simulink subsystem "low_level_mapper"  (R2020a)
settings: Solver=VariableStepAuto  StartTime=0.0  StopTime=10.0  RelTol=1e-3
values from neighbouring files (symbols this model uses):
  com_delay = 0.04    [init_conditions.m]
  g = 9.81    [init_conditions.m]
  m = (m_qc+0.006)*4 + m_main    (= 0.156)    [init_conditions.m]
undefined symbols (not defined in the file or in its folder): X, Y, Z
libraries: sm_lib x8, nesl_utility x8, simulink_extras x4
settings Model: Creator=Paul  LastModifiedBy=Paul

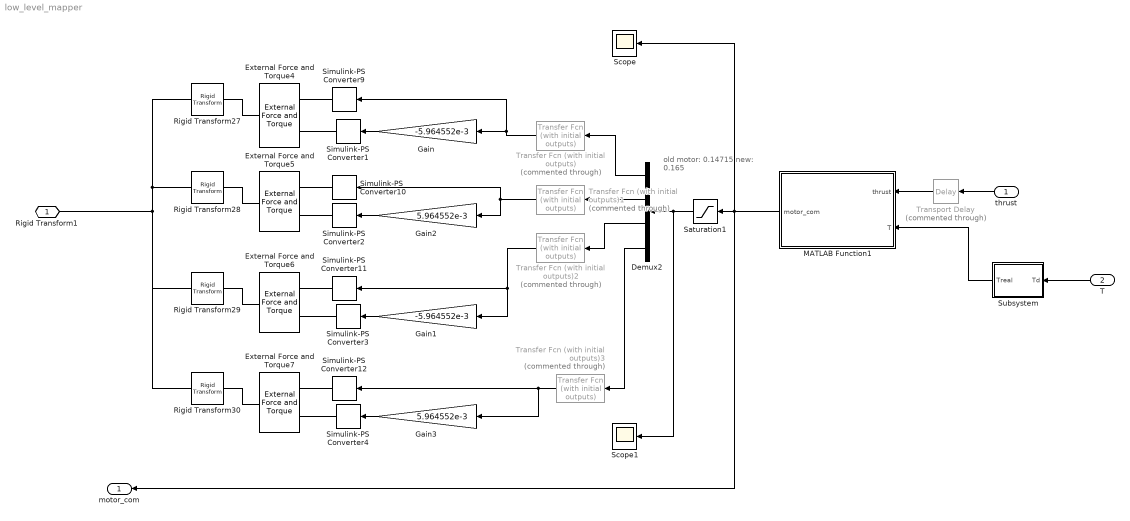
== system low_level_mapper ==
  note: old motor: 0.14715
      | new: 0.165
  thrust : Inport
  T : Inport  Port=2
  Demux2 : Demux
  External Force and Torque{4..7} (4 alike) : sm_lib/Forces and Torques/External Force and Torque  ForceResolutionFrame=AttachedFrame  EnableForceX=off  EnableForceY=off  EnableForceZ=on  EnableForce=off  TorqueResolutionFrame=AttachedFrame  EnableTorqueX=off  EnableTorqueY=off  EnableTorqueZ=on  EnableTorque=off
  Gain : Gain  Gain=-5.964552e-3
  Gain1 : Gain  Gain=-5.964552e-3
  Gain2 : Gain  Gain=5.964552e-3
  Gain3 : Gain  Gain=5.964552e-3
  MATLAB Function1 : MATLAB Function  TreatAsAtomicUnit=on
  Rigid Transform27 : sm_lib/Frames and Transforms/Rigid Transform  TranslationMethod=Cartesian  TranslationStandardOffset=0.4  TranslationLengthUnit=m  TranslationStandardAxis=+X  TranslationCartesianOffset=[0.03165 0.03165 0]  TranslationROffset=0  TranslationROffsetUnits=m  TranslationZOffset=0  TranslationZOffsetUnits=m  TranslationThetaOffset=0  TranslationThetaOffsetUnits=deg  RotationMethod=None  RotationAngleUnits=deg  RotationStandardAxis=+X  RotationAngle=90  RotationArbitraryAxis=[0 0 1]  FollAlignAxisA=+X  BaseAlignAxisA=+Y  FollAlignAxisB=+Y  BaseAlignAxisB=+Z  RotationSequenceAxes=FollowerAxes  RotationSequence=XYX  RotationSequenceAngles=[0 0 0]  RotationSequenceAnglesUnits=deg  RotationMatrix=[1 0 0; 0 1 0; 0 0 1]
  Rigid Transform28 : sm_lib/Frames and Transforms/Rigid Transform  TranslationMethod=Cartesian  TranslationStandardOffset=0.4  TranslationLengthUnit=m  TranslationStandardAxis=+X  TranslationCartesianOffset=[0.03165 -0.03165 0]  TranslationROffset=0  TranslationROffsetUnits=m  TranslationZOffset=0  TranslationZOffsetUnits=m  TranslationThetaOffset=0  TranslationThetaOffsetUnits=deg  RotationMethod=None  RotationAngleUnits=deg  RotationStandardAxis=+X  RotationAngle=90  RotationArbitraryAxis=[0 0 1]  FollAlignAxisA=+X  BaseAlignAxisA=+Y  FollAlignAxisB=+Y  BaseAlignAxisB=+Z  RotationSequenceAxes=FollowerAxes  RotationSequence=XYX  RotationSequenceAngles=[0 0 0]  RotationSequenceAnglesUnits=deg  RotationMatrix=[1 0 0; 0 1 0; 0 0 1]
  Rigid Transform29 : sm_lib/Frames and Transforms/Rigid Transform  TranslationMethod=Cartesian  TranslationStandardOffset=0.4  TranslationLengthUnit=m  TranslationStandardAxis=+X  TranslationCartesianOffset=[-0.03165 -0.03165 0]  TranslationROffset=0  TranslationROffsetUnits=m  TranslationZOffset=0  TranslationZOffsetUnits=m  TranslationThetaOffset=0  TranslationThetaOffsetUnits=deg  RotationMethod=None  RotationAngleUnits=deg  RotationStandardAxis=+X  RotationAngle=90  RotationArbitraryAxis=[0 0 1]  FollAlignAxisA=+X  BaseAlignAxisA=+Y  FollAlignAxisB=+Y  BaseAlignAxisB=+Z  RotationSequenceAxes=FollowerAxes  RotationSequence=XYX  RotationSequenceAngles=[0 0 0]  RotationSequenceAnglesUnits=deg  RotationMatrix=[1 0 0; 0 1 0; 0 0 1]
  Rigid Transform30 : sm_lib/Frames and Transforms/Rigid Transform  TranslationMethod=Cartesian  TranslationStandardOffset=0.4  TranslationLengthUnit=m  TranslationStandardAxis=+X  TranslationCartesianOffset=[-0.03165 0.03165 0]  TranslationROffset=0  TranslationROffsetUnits=m  TranslationZOffset=0  TranslationZOffsetUnits=m  TranslationThetaOffset=0  TranslationThetaOffsetUnits=deg  RotationMethod=None  RotationAngleUnits=deg  RotationStandardAxis=+X  RotationAngle=90  RotationArbitraryAxis=[0 0 1]  FollAlignAxisA=+X  BaseAlignAxisA=+Y  FollAlignAxisB=+Y  BaseAlignAxisB=+Z  RotationSequenceAxes=FollowerAxes  RotationSequence=XYX  RotationSequenceAngles=[0 0 0]  RotationSequenceAnglesUnits=deg  RotationMatrix=[1 0 0; 0 1 0; 0 0 1]
  Saturation1 : Saturate  UpperLimit=0.17  LowerLimit=0
  Scope : Scope
  Scope1 : Scope
  Simulink-PS Converter{1..4,9..12} (8 alike) : nesl_utility/Simulink-PS Converter  PhysicalDomain=network_engine_domain  SubClassName=ps_input  LeftPortType=input  RightPortType=output  PseudoPeriodic=off  Frequencies=[]  NoiseDistribution=none  NoiseParameters=[]  Unit=1  AffineConversion=off  FilteringAndDerivatives=zero  SimscapeFilterOrder=1  InputFilterTimeConstant=0.001  UdotUserProvided=0
  Subsystem : Subsystem
  Transfer Fcn (with initial outputs){,1..3} (4 alike) : simulink_extras/Additional Linear/Transfer Fcn (with initial outputs)  Commented=through  N=[1]  D="[0.02  1]"  Y0=0  U0=0
  Transport Delay : TransportDelay  Commented=through  DelayTime=com_delay  InitialOutput=m*g/4
  Rigid Transform1 : PMIOPort  Side=Right
  motor_com : Outport
  wires:
  T/1 -> Subsystem/1(Td)
  Demux2/4 -> Transfer Fcn (with initial outputs)3/1
  MATLAB Function1/1(motor_com) -> Saturation1/1, Scope/1, motor_com/1
  Demux2/1 -> Transfer Fcn (with initial outputs)/1
  Demux2/2 -> Transfer Fcn (with initial outputs)1/1
  Saturation1/1 -> Demux2/1, Scope1/1
  Demux2/3 -> Transfer Fcn (with initial outputs)2/1
  thrust/1 -> Transport Delay/1
  Transport Delay/1 -> MATLAB Function1/1(thrust)
  Subsystem/1(Treal) -> MATLAB Function1/2(T)
  Gain/1 -> Simulink-PS Converter1/1
  Gain1/1 -> Simulink-PS Converter3/1
  Gain2/1 -> Simulink-PS Converter2/1
  Gain3/1 -> Simulink-PS Converter4/1
  Transfer Fcn (with initial outputs)/1 -> Gain/1, Simulink-PS Converter9/1
  Transfer Fcn (with initial outputs)1/1 -> Simulink-PS Converter10/1, Gain2/1
  Transfer Fcn (with initial outputs)2/1 -> Simulink-PS Converter11/1, Gain1/1
  Transfer Fcn (with initial outputs)3/1 -> Simulink-PS Converter12/1, Gain3/1
  connections:
  Rigid Transform27/LConn1 -- Rigid Transform29/LConn1 -- Rigid Transform30/LConn1 -- Rigid Transform1/RConn1 -- Rigid Transform28/LConn1
  Simulink-PS Converter9/RConn1 -- External Force and Torque4/LConn1
  Simulink-PS Converter11/RConn1 -- External Force and Torque6/LConn1
  External Force and Torque4/RConn1 -- Rigid Transform27/RConn1
  External Force and Torque6/RConn1 -- Rigid Transform29/RConn1
  Simulink-PS Converter10/RConn1 -- External Force and Torque5/LConn1
  Simulink-PS Converter12/RConn1 -- External Force and Torque7/LConn1
  Rigid Transform30/RConn1 -- External Force and Torque7/RConn1
  Rigid Transform28/RConn1 -- External Force and Torque5/RConn1
  Simulink-PS Converter1/RConn1 -- External Force and Torque4/LConn2
  Simulink-PS Converter2/RConn1 -- External Force and Torque5/LConn2
  Simulink-PS Converter3/RConn1 -- External Force and Torque6/LConn2
  Simulink-PS Converter4/RConn1 -- External Force and Torque7/LConn2

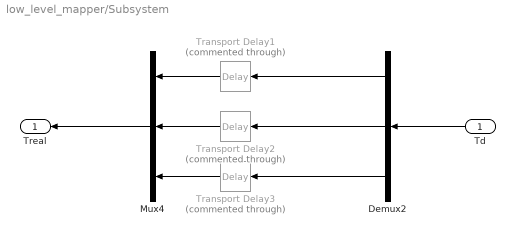
== system low_level_mapper/Subsystem ==
  Td : Inport
  Demux2 : Demux  Outputs=3
  Mux4 : Mux  Inputs=3
  Transport Delay1 : TransportDelay  Commented=through  DelayTime=com_delay
  Transport Delay2 : TransportDelay  Commented=through  DelayTime=com_delay
  Transport Delay3 : TransportDelay  Commented=through  DelayTime=com_delay
  Treal : Outport  VectorParamsAs1DForOutWhenUnconnected=off
  wires:
  Transport Delay3/1 -> Mux4/3
  Transport Delay2/1 -> Mux4/2
  Transport Delay1/1 -> Mux4/1
  Td/1 -> Demux2/1
  Mux4/1 -> Treal/1
  Demux2/3 -> Transport Delay3/1
  Demux2/1 -> Transport Delay1/1
  Demux2/2 -> Transport Delay2/1

== matlab function low_level_mapper/MATLAB Function1 ==
  data: thrust input; T input; motor_com output
function motor_com = combine(thrust, T)

% force and moment contribution by single blade
thrust = thrust/4;
tx = T(1)/4;
ty = T(2)/4;
tz = T(3)/4;

ftx = tx/(31.64e-3);
fty = ty/(31.64e-3);
ftz = tz/(31.64e-3) * 5.3; % determined by c_p and c_t

f0 = thrust + ftx - fty - ftz;
f1 = thrust - ftx - fty + ftz;
f2 = thrust - ftx + fty - ftz;
f3 = thrust + ftx + fty + ftz;


% % 0.015kg * 9.81 = 0.1472
% actual motor command in Crazyflie firmware
% m0 = (-0.06767+sqrt(0.06767^2+4*0.0915*f0))/(2*0.0915) * 65535;
% m1 = (-0.06767+sqrt(0.06767^2+4*0.0915*f1))/(2*0.0915) * 65535;
% m2 = (-0.06767+sqrt(0.06767^2+4*0.0915*f2))/(2*0.0915) * 65535;
% m3 = (-0.06767+sqrt(0.06767^2+4*0.0915*f3))/(2*0.0915) * 65535;

motor_com = [f0;f1;f2;f3];
